simulink model "Lateral_Autopilot_Jetstar_FC4_Testing_Linear_Model"  (R2020a)
settings: Solver=FixedStepAuto  StartTime=0.0  StopTime=30  FixedStep=0.01  RelTol=1e-3
model workspace: external: MAT-File E:\Autopilot\Task 6\GP04_Task6_Codes\Lateral_Matrices.mat (data not in the file)
values from neighbouring files (symbols this model uses):
  A_Lat = [Yv        ,   Yp+w_0    ,   Yr-u_0         ,   g*cos(theta_0)   ,   0 ... (first row only)    [Lateral_Linearized_Matrices.m]    (also in Lateral_Matrices.mat = [-0.229 -0.0124232081911 0.00933447098976 0 0 27.6043801159 )
  B_Lat = [0             ,    Ydel_r ... (first row only)    [Lateral_Linearized_Matrices.m]    (also in Lateral_Matrices.mat = [0  32.6402; 5.71  2.77; -0.0524  -3.12; 0  0; 0  0])
  C_Lat = eye(5)    [Lateral_Linearized_Matrices.m]    (also in Lateral_Matrices.mat = [1 0 0 0 0 0 1 0 0 0 0 0 ... (25 elements, 5x5)])
  D_Lat = zeros(5,2)    [Lateral_Linearized_Matrices.m]    (also in Lateral_Matrices.mat = [0  0; 0  0; 0  0; 0  0; 0  0])
  g = 32.17405    [Lateral_Matrices.mat]    (also in ReadExcelModified.m = aircraft_data(52))
  u_0 = 585.349466728    [Lateral_Matrices.mat]    (also in ReadExcelModified.m = s0(1))
  Vto = 586    [Lateral_Matrices.mat]    (also in ReadExcelModified.m = sqrt(s0(1)^2 + s0(2)^2 + s0(3)^2))
libraries: simulink_extras x4
settings Model: Creator=mohan  LastModifiedBy=mohan

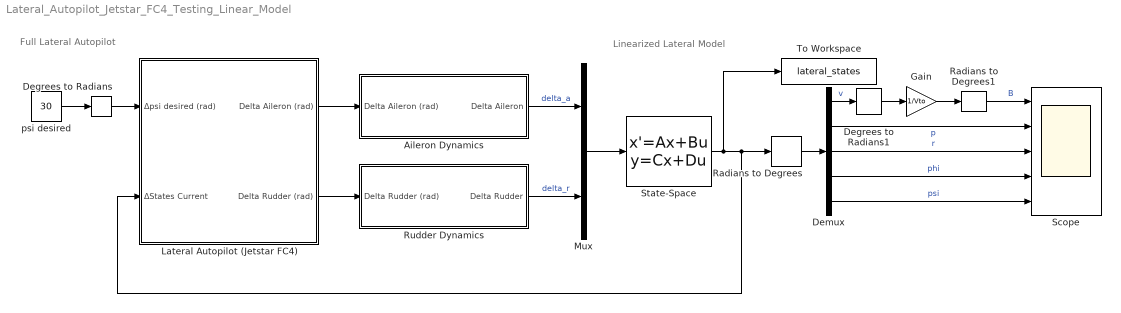
== system Lateral_Autopilot_Jetstar_FC4_Testing_Linear_Model ==
  note: Linearized Lateral Model
  note: Full Lateral Autopilot
  Aileron Dynamics : Subsystem  mask{delta_a_max=50}
      mask prompts: delta_a_max "Maximum Aileron Deflection (deg)"
      mask DialogControl ParameterGroupVar Prompt: Rudder Limits
  Degrees to Radians : simulink_extras/Transformations/Degrees to Radians
  Degrees to Radians1 : simulink_extras/Transformations/Degrees to Radians
  Demux : Demux  Outputs=5
  Gain : Gain  Gain=1/Vto
  Lateral Autopilot (Jetstar FC4) : Subsystem  mask{Kp_yaw=0.38326, taw_HPF=1/0.7, Kp_roll=1.0063, Kd_roll=0.32967, taw_coordination=20}
      mask prompts: Kp_yaw "Kp"; taw_HPF "Taw (Washout)"; Kp_roll "Kp"; Kd_roll "Kd"; taw_coordination "Taw"
      mask DialogControl ParameterGroupVar Prompt: Controllers
      mask DialogControl Container4 Prompt: Yaw Damper Gains (P + Washout)
      mask DialogControl Container5 Prompt: Roll Controller (PD)
      mask DialogControl Container6 Prompt: Coordinated Turn
  Mux : Mux  Inputs=2
  Radians to Degrees : simulink_extras/Transformations/Radians to Degrees
  Radians to Degrees1 : simulink_extras/Transformations/Radians to Degrees
  Rudder Dynamics : Subsystem  mask{delta_r_max=25}
      mask prompts: delta_r_max "Maximum Rudder Deflection (deg)"
      mask DialogControl ParameterGroupVar Prompt: Rudder Limits
  Scope : Scope  NumInputPorts=5
  State-Space : StateSpace  A=A_Lat  B=B_Lat  C=C_Lat  D=D_Lat  InitialCondition=0
  To Workspace : ToWorkspace  VariableName=lateral_states  SaveFormat=Timeseries  SampleTime=-1
  psi desired : Constant  Value=30
  wires:
  Mux/1 -> State-Space/1
  State-Space/1 -> To Workspace/1, Lateral Autopilot (Jetstar FC4)/2(ΔStates Current), Radians to Degrees/1
  Demux/1 -> Degrees to Radians1/1  "v"
  Demux/2 -> Scope/2  "p"
  Demux/3 -> Scope/3  "r"
  Demux/4 -> Scope/4  "phi"
  Demux/5 -> Scope/5  "psi"
  Radians to Degrees/1 -> Demux/1
  Lateral Autopilot (Jetstar FC4)/1(Delta Aileron (rad)) -> Aileron Dynamics/1(Delta Aileron (rad))
  Rudder Dynamics/1(Delta Rudder) -> Mux/2  "delta_r"
  Lateral Autopilot (Jetstar FC4)/2(Delta Rudder (rad)) -> Rudder Dynamics/1(Delta Rudder (rad))
  Aileron Dynamics/1(Delta Aileron) -> Mux/1  "delta_a"
  psi desired/1 -> Degrees to Radians/1
  Degrees to Radians/1 -> Lateral Autopilot (Jetstar FC4)/1(Δpsi desired (rad))
  Degrees to Radians1/1 -> Gain/1
  Gain/1 -> Radians to Degrees1/1
  Radians to Degrees1/1 -> Scope/1  "B"

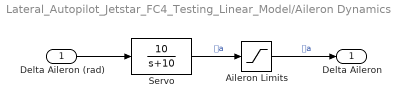
== system Lateral_Autopilot_Jetstar_FC4_Testing_Linear_Model/Aileron Dynamics ==
  Delta Aileron (rad) : Inport
  Aileron Limits : Saturate  UpperLimit=delta_a_max*pi/180  LowerLimit=-delta_a_max*pi/180
  Servo : TransferFcn  Numerator=[10]  Denominator=[1 10]
  Delta Aileron : Outport
  wires:
  Servo/1 -> Aileron Limits/1  "𝛿a"
  Aileron Limits/1 -> Delta Aileron/1  "𝛿a"
  Delta Aileron (rad)/1 -> Servo/1

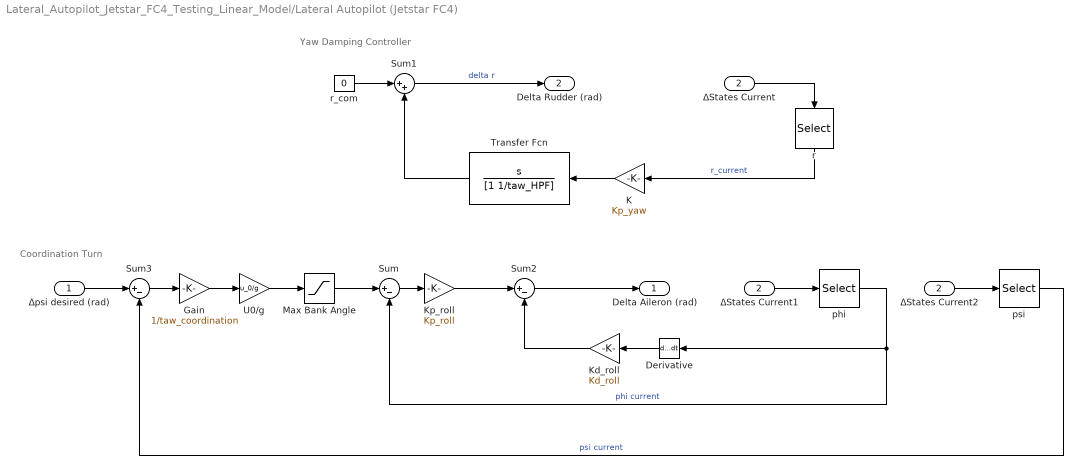
== system Lateral_Autopilot_Jetstar_FC4_Testing_Linear_Model/Lateral Autopilot (Jetstar FC4) ==
  note: Coordination Turn
  note: Yaw Damping Controller
  Δpsi desired (rad) : Inport
  ΔStates Current : Inport  Port=2
  Derivative : Derivative
  Gain : Gain  Gain=1/taw_coordination
  K : Gain  Gain=Kp_yaw
  Kd_roll : Gain  Gain=Kd_roll
  Kp_roll : Gain  Gain=Kp_roll
  Max Bank Angle : Saturate  UpperLimit=30*pi/180  LowerLimit=-30*pi/180
  Sum : Sum  Inputs=|+-
  Sum1 : Sum  Inputs=|++
  Sum2 : Sum  Inputs=|+-
  Sum3 : Sum  Inputs=|+-
  Transfer Fcn : TransferFcn  Numerator=[1 0]  Denominator=[1 1/taw_HPF]
  U0/g : Gain  Gain=u_0/g
  phi : Selector  InputPortWidth=5  IndexOptions=Index vector (dialog)  Indices=4  OutputSizes=1
  psi : Selector  InputPortWidth=5  IndexOptions=Index vector (dialog)  Indices=5  OutputSizes=1
  r : Selector  InputPortWidth=5  IndexOptions=Index vector (dialog)  Indices=3  OutputSizes=1
  r_com : Constant  Value=0
  ΔStates Current1 : InportShadow  Port=2
  ΔStates Current2 : InportShadow  Port=2
  Delta Aileron (rad) : Outport
  Delta Rudder (rad) : Outport  Port=2
  wires:
  r/1 -> K/1  "r_current"
  r_com/1 -> Sum1/1
  Transfer Fcn/1 -> Sum1/2
  K/1 -> Transfer Fcn/1
  Sum1/1 -> Delta Rudder (rad)/1  "delta r"
  ΔStates Current/1 -> r/1
  ΔStates Current1/1 -> phi/1
  Sum/1 -> Kp_roll/1
  Kd_roll/1 -> Sum2/2
  Sum2/1 -> Delta Aileron (rad)/1
  phi/1 -> Derivative/1, Sum/2  "phi current"
  Derivative/1 -> Kd_roll/1
  Kp_roll/1 -> Sum2/1
  Max Bank Angle/1 -> Sum/1
  Δpsi desired (rad)/1 -> Sum3/1
  ΔStates Current2/1 -> psi/1
  psi/1 -> Sum3/2  "psi current"
  Sum3/1 -> Gain/1
  U0/g/1 -> Max Bank Angle/1
  Gain/1 -> U0/g/1

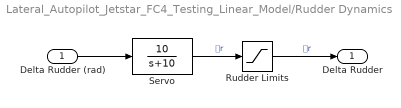
== system Lateral_Autopilot_Jetstar_FC4_Testing_Linear_Model/Rudder Dynamics ==
  Delta Rudder (rad) : Inport
  Rudder Limits : Saturate  UpperLimit=delta_r_max*pi/180  LowerLimit=-delta_r_max*pi/180
  Servo : TransferFcn  Numerator=[10]  Denominator=[1 10]
  Delta Rudder : Outport
  wires:
  Servo/1 -> Rudder Limits/1  "𝛿r"
  Rudder Limits/1 -> Delta Rudder/1  "𝛿r"
  Delta Rudder (rad)/1 -> Servo/1
